simulink model "torque_balance_controller"  (R2022a)
settings: Solver=VariableStepAuto  StartTime=0.0  StopTime=4  MaxStep=0.01  RelTol=1e-3
values from neighbouring files (symbols this model uses):
  k_gn = m*g/0.001    (= 412020)    [controller_parameters.m]
  k_gt = m*g/0.1    (= 4120.2)    [controller_parameters.m]
  m = 42    [controller_parameters.m]    (also in ground_reaction_params.m = 12)
  mu_slide = 0.8    [controller_parameters.m]    (also in ground_reaction_params.m = 0.008)
  mu_stick = 0.9    [controller_parameters.m]    (also in ground_reaction_params.m = 0.009)
  v_gn_max = 0.03    [controller_parameters.m]
  v_gt_max = 0.03    [controller_parameters.m]
  vLimit = 0.01    [controller_parameters.m]    (also in ground_reaction_params.m = 0.001)
undefined symbols (not defined in the file or in its folder): Newton, Raphson, X, Y, Z
libraries: sm_lib x179, nesl_utility x110, simulink x32, simulink_extras x8
(part 1 of 8)
settings Model: Creator=nemo  LastModifiedBy=nemo

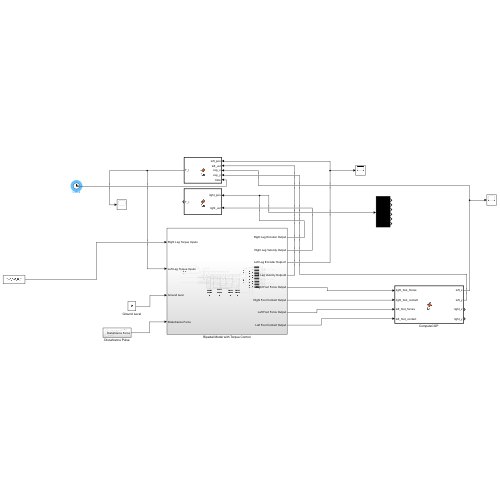
[thumbnail: Simulink's stored preview of the top-level diagram]
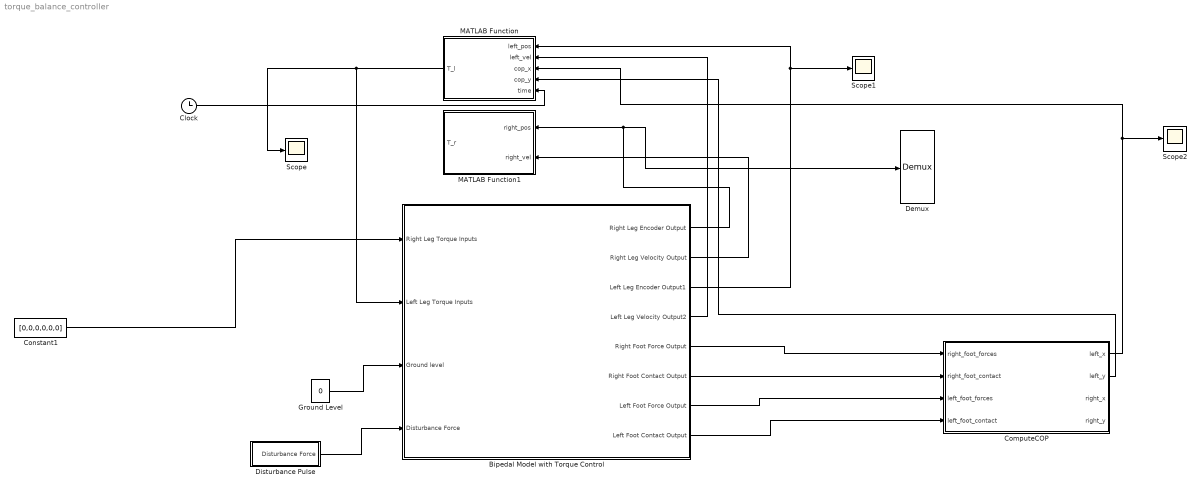
== system torque_balance_controller ==
  Bipedal Model with Torque Control : Subsystem
  Clock : Clock
  "ComputeCOP " : MATLAB Function  TreatAsAtomicUnit=on
  Constant1 : Constant  Value=[0,0,0,0,0,0]
  Demux : Demux  Outputs=6
  Disturbance Pulse : Subsystem
  Ground Level : Constant  Value=0
  MATLAB Function : MATLAB Function  TreatAsAtomicUnit=on
  MATLAB Function1 : MATLAB Function  TreatAsAtomicUnit=on
  Scope : Scope
  Scope1 : Scope
  Scope2 : Scope
  wires:
  Disturbance Pulse/1(Disturbance Force) -> Bipedal Model with Torque Control/4(Disturbance Force)
  Ground Level/1 -> Bipedal Model with Torque Control/3(Ground level)
  Bipedal Model with Torque Control/5(Right Foot Force Output) -> "ComputeCOP "/1(right_foot_forces)
  Bipedal Model with Torque Control/6(Right Foot Contact Output) -> "ComputeCOP "/2(right_foot_contact)
  Bipedal Model with Torque Control/8(Left Foot Contact Output) -> "ComputeCOP "/4(left_foot_contact)
  Bipedal Model with Torque Control/7(Left Foot Force Output) -> "ComputeCOP "/3(left_foot_forces)
  Bipedal Model with Torque Control/3(Left Leg Encoder Output1) -> MATLAB Function/1(left_pos), Scope1/1
  Bipedal Model with Torque Control/4(Left Leg Velocity Output2) -> MATLAB Function/2(left_vel)
  Bipedal Model with Torque Control/1(Right Leg Encoder Output) -> MATLAB Function1/1(right_pos), Demux/1
  Bipedal Model with Torque Control/2(Right Leg Velocity Output) -> MATLAB Function1/2(right_vel)
  Constant1/1 -> Bipedal Model with Torque Control/1(Right Leg Torque Inputs)
  MATLAB Function/1(T_l) -> Bipedal Model with Torque Control/2(Left Leg Torque Inputs), Scope/1
  "ComputeCOP "/1(left_x) -> Scope2/1, MATLAB Function/3(cop_x)
  "ComputeCOP "/2(left_y) -> MATLAB Function/4(cop_y)
  Clock/1 -> MATLAB Function/5(time)
